simulink model "G29_test"  (R2024b)
settings: Solver=FixedStepAuto  StartTime=0.0  StopTime=inf  RelTol=1e-3
values from neighbouring files (symbols this model uses):
  G29 = struct    [model2_dim.m]    (also in model2_dim_Chikri.m)
libraries: slrealtimeG29lib x1
settings Model: Creator=simulatorATM  LastModifiedBy=simulatorATM
settings SolverCC: ConcurrentTasks=on  PositivePriorityOrder=on
settings OptimizationCC: BlockReduction=off  OptimizeBlockIOStorage=off
settings DebuggingCC: TasksWithSamePriorityMsg=none
settings HardwareCC: ProdBitPerLong=64  ProdLongLongMode=on  ProdHWDeviceType=Intel->x86-64 (Linux 64)
settings RTWCC: Description=Speedgoat Real-Time Target Machine  SystemTargetFile=speedgoat.tlc  TemplateMakefile=slrealtime_default_tmf  Toolchain=Simulink Real-Time Toolchain  BuildConfiguration=Faster Runs  CodeExecutionProfiling=on  TargetLang=C++
settings SimulinkRealTimeTargetCC: InstructionSetFMA=off  LogToMDFFile=off

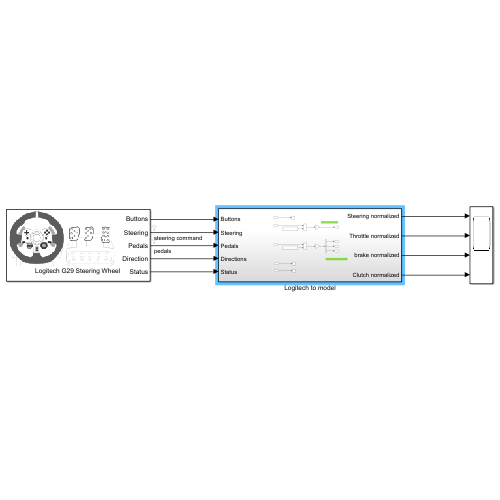
[thumbnail: Simulink's stored preview of the top-level diagram]
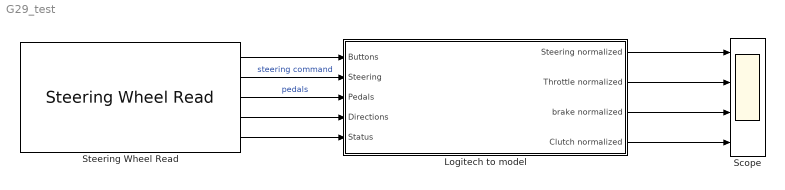
== system G29_test ==
  Logitech to model : Subsystem
  Scope : Scope  NumInputPorts=4
  Steering Wheel Read : slrealtimeG29lib/Steering Wheel Read  sampleTime=-1
  wires:
  Steering Wheel Read/1 -> Logitech to model/1(Buttons)
  Steering Wheel Read/2 -> Logitech to model/2(Steering)  "steering command"
  Steering Wheel Read/3 -> Logitech to model/3(Pedals)  "pedals"
  Steering Wheel Read/4 -> Logitech to model/4(Directions)
  Steering Wheel Read/5 -> Logitech to model/5(Status)
  Logitech to model/1(Steering normalized) -> Scope/1
  Logitech to model/2(Throttle normalized) -> Scope/2
  Logitech to model/3(brake normalized) -> Scope/3
  Logitech to model/4(Clutch normalized) -> Scope/4

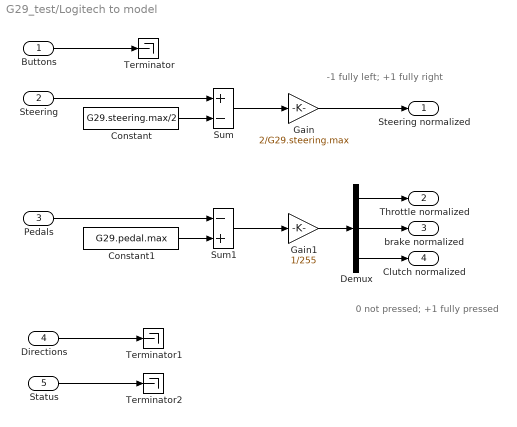
== system G29_test/Logitech to model ==
  note: -1 fully left; +1 fully right
  note: 0 not pressed; +1 fully pressed
  Buttons : Inport
  Steering : Inport  Port=2
  Pedals : Inport  Port=3
  Directions : Inport  Port=4
  Status : Inport  Port=5
  Constant : Constant  Value=G29.steering.max/2
  Constant1 : Constant  Value=G29.pedal.max
  Demux : Demux  Outputs=3
  Gain : Gain  Gain=2/G29.steering.max
  Gain1 : Gain  Gain=1/255
  Sum : Sum  Inputs=+-
  Sum1 : Sum  Inputs=-+
  Terminator : Terminator
  Terminator1 : Terminator
  Terminator2 : Terminator
  Steering normalized : Outport
  Throttle normalized : Outport  Port=2
  brake normalized : Outport  Port=3
  Clutch normalized : Outport  Port=4
  wires:
  Buttons/1 -> Terminator/1
  Directions/1 -> Terminator1/1
  Status/1 -> Terminator2/1
  Steering/1 -> Sum/1
  Sum/1 -> Gain/1
  Constant/1 -> Sum/2
  Gain/1 -> Steering normalized/1
  Sum1/1 -> Gain1/1
  Pedals/1 -> Sum1/1
  Constant1/1 -> Sum1/2
  Gain1/1 -> Demux/1
  Demux/1 -> Throttle normalized/1
  Demux/2 -> brake normalized/1
  Demux/3 -> Clutch normalized/1
